simulink model "Controller_obstacle"  (R2024a)
settings: Solver=FixedStepAuto  StartTime=0.0  StopTime=10.0  FixedStep=Ts  MaxStep=Ts  RelTol=1e-3
libraries: slpidlib x1
settings Model: DataDictionary=data_interface.sldd  Creator=upattacini  LastModifiedBy=amelis
settings DataIOCC: SaveOutput=off  DSMLogging=off  SaveTime=off  ReturnWorkspaceOutputs=off
settings ModelReferenceCC: ModelReferenceNumInstancesAllowed=Single
settings RTWCC: GPUComputeCapability=3.5

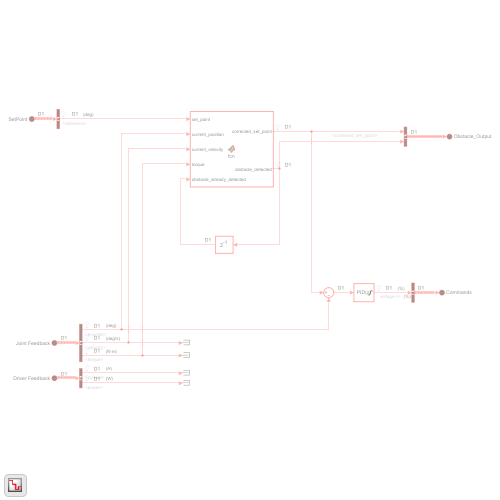
[thumbnail: Simulink's stored preview of the top-level diagram]
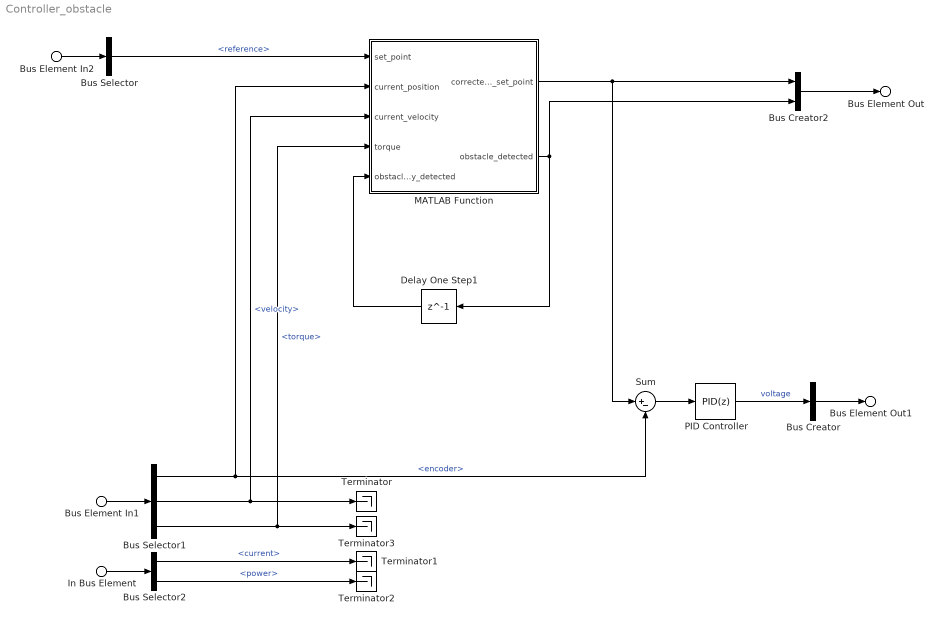
== system Controller_obstacle ==
  Bus Element In2 : Inport  PortName=SetPoint
  Bus Element In1 : Inport  Port=2  PortName=Joint Feedback
  In Bus Element : Inport  Port=3  PortName=Driver Feedback
  Bus Creator : BusCreator  Inputs=1  OutDataTypeStr=Bus: Control_Command  NonVirtualBus=on
      settings: InheritFromInputs=off
  Bus Creator2 : BusCreator  Inputs=2
  Bus Selector : BusSelector  OutputSignals=reference
  Bus Selector1 : BusSelector  OutputSignals=encoder,velocity,torque
  Bus Selector2 : BusSelector  OutputSignals=current,power
  Delay One Step1 : Delay  DelayLength=1
  MATLAB Function : MATLAB Function  TreatAsAtomicUnit=on
  PID Controller : slpidlib/PID Controller  Controller=PID  Form=Parallel  TimeDomain=Discrete-time  UseExternalTs=off  SampleTime=-1  IntegratorMethod=Trapezoidal  FilterMethod=Forward Euler  ControllerParametersSource=internal  P=2  I=0.4  UseKiTs=off  D=0.03  UseExternalDerivativeSource=off  N=100  UseFilter=on  TunerSelectOption=Transfer Function Based (PID Tuner App)  InitialConditionSource=internal  InitialConditionForIntegrator=0  InitialConditionForFilter=0  DifferentiatorICPrevScaledInput=0  ExternalReset=none  TrackingMode=off  Kt=1  LimitOutput=on  SatLimitsSource=internal  UpperSaturationLimit=100  LowerSaturationLimit=-100  LinearizeAsGain=on  AntiWindupMode=clamping  Kb=1  LimitIntegrator=off  UpperIntegratorSaturationLimit=inf  LowerIntegratorSaturationLimit=-inf  POutMin=[]  POutMax=[]  IOutMin=[]  IOutMax=[]  DOutMin=[]  DOutMax=[]  NOutMin=[]  NOutMax=[]  SumOutMin=[]  SumOutMax=[]  SaturationOutMin=[]  SaturationOutMax=[]  PParamMin=[]  PParamMax=[]  IParamMin=[]  IParamMax=[]  DParamMin=[]  DParamMax=[]  NParamMin=[]  NParamMax=[]  KbParamMin=[]  KbParamMax=[]  KtParamMin=[]  KtParamMax=[]  KbOutMin=[]  KbOutMax=[]  KtOutMin=[]  KtOutMax=[]  IntegratorOutMin=[]  IntegratorOutMax=[]  FilterOutMin=[]  FilterOutMax=[]  SumI1OutMin=[]  SumI1OutMax=[]  SumI2OutMin=[]  SumI2OutMax=[]  SumI3OutMin=[]  SumI3OutMax=[]  SumI4OutMin=[]  SumI4OutMax=[]  SumDOutMin=[]  SumDOutMax=[]  DifferentiatorOutMin=[]  DifferentiatorOutMax=[]  FilterDiffOutCoefMin=[]  FilterDiffOutCoefMax=[]  ReciprocalOutMin=[]  ReciprocalOutMax=[]  SumDenOutMin=[]  SumDenOutMax=[]  SumNumOutMin=[]  SumNumOutMax=[]  DivideOutMin=[]  DivideOutMax=[]  UdiffTsProdOutMin=[]  UdiffTsProdOutMax=[]  NTsProdOutMin=[]  NTsProdOutMax=[]  UintegralTsProdOutMin=[]  UintegralTsProdOutMax=[]  UngainTsProdOutMin=[]  UngainTsProdOutMax=[]  ClampingZeroOutDataTypeStr=Inherit: Inherit via back propagation  ClampingZeroOutMin=[]  ClampingZeroOutMax=[]  FilterDenConstantOutDataTypeStr=Inherit: Inherit via back propagation  FilterDenConstantOutMin=[]  FilterDenConstantOutMax=[]  PCopyOutDataTypeStr=Inherit: Inherit via back propagation  PCopyOutMin=[]  PCopyOutMax=[]  NCopyOutDataTypeStr=Inherit: Inherit via back propagation  NCopyOutMin=[]  NCopyOutMax=[]  IntegratorContinuousStateAttributes=''  IntegratorStateMustResolveToSignalObject=off  IntegratorRTWStateStorageClass=Auto  FilterContinuousStateAttributes=''  FilterStateMustResolveToSignalObject=off  FilterRTWStateStorageClass=Auto  ParallelPVariant=InternalParameters  IdealPVariant=Disabled  IVariant=InternalParameters  DVariant=InternalParameters  IntegratorVariant=Discrete  SatVariant=Enabled  AWVariant=DiscClampingParallel  PCopyVariant=Disabled  TRVariant=Disabled  FdbkBlocksVariant=Feedback  IdealPFdbkVariant=Passthrough  SatFdbkVariant=Passthrough  DerivativeFilterVariant=ForwardEulerFilter  NVariant=InternalParameters  NCopyVariant=Disabled  FilterICVariant=InternalICsFilter  IntegratorICVariant=InternalICs  ExternalResetVariant=Disabled  TRSumVariant=Passthrough  SumFdbkVariant=Enabled  SumVariant=Sum_PID  TsampFilterVariant=InternalTs  TsampNgainVariant=Passthrough  TsampIntegralVariant=Disabled_SignalSpec  ExternalSaturationOutDataTypeStr=Inherit: Same as second input  DerivativeSourceVariant=ErrorSignal
  Sum : Sum  Inputs=|+-
  Terminator{,1..3} (4 alike) : Terminator
  Bus Element Out1 : Outport  PortName=Commands
  Bus Element Out : Outport  Port=2  PortName=Obstacle_Output
  wires:
  Bus Creator/1 -> Bus Element Out1/1
  Bus Element In2/1 -> Bus Selector/1
  Sum/1 -> PID Controller/1
  Bus Selector1/2 -> MATLAB Function/3(current_velocity), Terminator/1  "<velocity>"
  Bus Selector2/2 -> Terminator2/1  "<power>"
  Bus Selector2/1 -> Terminator1/1  "<current>"
  In Bus Element/1 -> Bus Selector2/1
  Bus Selector1/3 -> MATLAB Function/4(torque), Terminator3/1  "<torque>"
  Bus Element In1/1 -> Bus Selector1/1
  PID Controller/1 -> Bus Creator/1  "voltage"
  Bus Creator2/1 -> Bus Element Out/1
  Bus Selector/1 -> MATLAB Function/1(set_point)  "<reference>"
  Bus Selector1/1 -> Sum/2, MATLAB Function/2(current_position)  "<encoder>"
  MATLAB Function/2(obstacle_detected) -> Bus Creator2/2, Delay One Step1/1
  Delay One Step1/1 -> MATLAB Function/5(obstacle_already_detected)
  MATLAB Function/1(corrected_set_point) -> Sum/1, Bus Creator2/1

== matlab function Controller_obstacle/MATLAB Function ==
  data: set_point input; current_position input; current_velocity input; torque input; obstacle_already_detected input; corrected_set_point output; obstacle_detected output
function [corrected_set_point, obstacle_detected] = fcn(set_point, current_position, current_velocity, torque, obstacle_already_detected)

max_settling_velocity = 2;

% safety bound includes unmodelled dynamics, like friction, and a safety
% coefficient

safety_bound = 1; % Nm
pendulum_mass = 0.1; % Kg
pendulum_1_lenght = 0.2; % m
g = 9.81; % m/s^2

gravity_torque = -pendulum_mass*g*(pendulum_1_lenght/2)*sind(current_position);
torque_bound = abs(gravity_torque) + safety_bound;

% Obstacle detection

if((abs(current_velocity) < max_settling_velocity && abs(torque) > torque_bound && obstacle_already_detected == 0) || obstacle_already_detected == 1)
    obstacle_detected = 1;
else
    obstacle_detected = 0;
end

% Reduce force to less than 1N in 1s

k_1 = 0.1;
minimum_contact_force = 0.1;

force_applied = (torque - gravity_torque)/pendulum_1_lenght; % not considering friction

% the set point in case of obstacle contact is equal to the current
% position (so that is subtracted then in the error computation) and an
% error term proportional to the force applied minus a minimum contact
% force considered
correction_term = current_position + k_1*(sign(force_applied)*(abs(force_applied)-minimum_contact_force));

% Stop new setpoints

if (obstacle_detected)
    corrected_set_point = correction_term;
else
    corrected_set_point = set_point;
end
